simulink library "commutil"  (Simulink 5.0)
values from neighbouring files (symbols this model uses):
  En = get_param(block, 'maskenables')    [commblkawgnchan.m]    (also in commblkbernoullisrc.m; commblkdemap.m; commblkdrpt.m; commblkeyescatdisc.m = get_param(block, 'MaskEnables'))
  IPValues = (0:M-1)    [commblkdemap.m]    (also in commblkmap.m)
  OPValues = MapVec    [commblkdemap.m]    (also in commblkmap.m)
undefined symbols (not defined in the file or in its folder): SatValue
libraries: commutil x8, dsparch2 x1, dspswit2 x1
settings Model: RequirementInfo=9  Creator=tdelve  LastModifiedBy=mmclerno

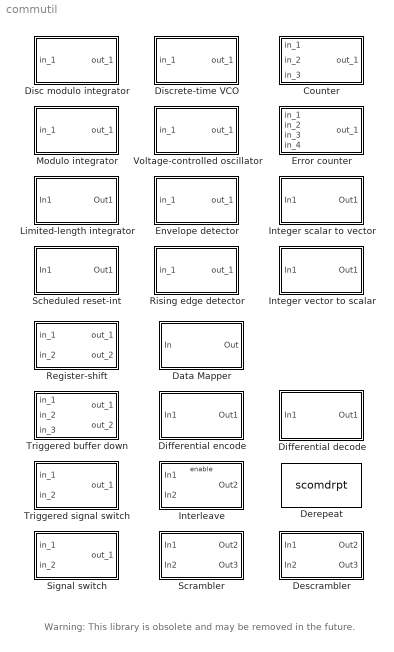
== system commutil ==
  note: Warning:  This library is obsolete and may be
      | removed in the future.
  Counter : Subsystem  mask(Resettable number counter){thld=.2}
      mask prompts: thld "Threshold:"
      mask help: If the 1st inport value is larger than the threshold, the counter increases one at the rising edge of the 2nd inport pulse.
      mask Help: If the signal at the 1st inport is larger than or equal to the given threshold at the rising edge of the 2nd inport, the counter increases by one. The rising edge of the 3rd port resets the counter to zero.
      mask Display:
      | plot(0,0,100,100,[5 10 10 8 10 12 10 10 15],[5 5 12 8 12 8 12 15 15]+40,[5 10 10 8 10 12 10 10 15],[5 5 12 8 12 8 12 15 15]);
      | disp('Counter')
  Data Mapper : Subsystem  mask(Data Mapper){MapMode=Binary to Gray, M=8, MapVec=[0 1 3 2 7 6 4 5]}
      mask prompts: MapMode "Mapping mode:"; M "Symbol set size (M):"; MapVec "Mapping vector:"
      mask help: Map integer symbols from one coding scheme to another.
      mask init:
      | [En,IPValues,OPValues,SatValue]=commblkmapdata(gcb,'init',{MapMode M MapVec});
      mask Help:
      | <P><FONT SIZE=+0>The Data Mapper block accepts integer inputs and produces
      | integer outputs. You can select one of four mapping modes: <B>Binary to
      | Gray, Gray to Binary, User Defined, or Straight Through</B>.</FONT>
      | 
      | <P><FONT SIZE=+0>Gray coding is an ordering of binary numbers such that
      | all adjacent numbers differ by only one bit. However, the inputs and outputs
      | of this block are integers, not binary vectors. As a result, the first
      | two mapping modes perform code conversions as follows:</FONT>
      | <UL type="disc">
      | <LI>
      | <FONT SIZE=+0>In the <B>Binary to Gray</B> mode, the output from this block
      | is the integer equivalent of the Gray code bit representation for the input
      | integer.</FONT></LI>
      | 
      | <LI>
      | <FONT SIZE=+0>In the <B>Gray to Binary</B> mode, the output from this block
      | is the integer position of the binary equivalent of the input integer in
      | a Gray code ordering.</FONT></LI>
      | </UL>
      | <FONT SIZE=+0>As an example, the table below shows both the <B>Binary to
      | Gray</B> and <B>Gray to Binary</B> mappings for integers in the range 0
      | to 7.</FONT>
      | <BR>&nbsp;
      | <TABLE BORDER CELLPADDING=9 WIDTH="480" >
      | <TR>
      | <TD COLSPAN="4"><B><FONT SIZE=+0>Table 1: Example of Binary to Gray and
      | Gray to Binary Mappings</FONT></B></TD>
      | </TR>
      | 
      | <TR>
      | <TD COLSPAN="2" WIDTH="50%">
      | <CENTER><B><FONT SIZE=+0>Binary to Gray Mode</FONT></B></CENTER>
      | </TD>
      | 
      | <TD COLSPAN="2" WIDTH="50%">
      | <CENTER><B><FONT SIZE=+0>Gray to Binary Mode</FONT></B></CENTER>
      | </TD>
      | </TR>
      | 
      | <TR>
      | <TD WIDTH="25%">
      | <CENTER><B><FONT SIZE=+0>Input</FONT></B></CENTER>
      | </TD>
      | 
      | <TD WIDTH="25%">
      | <CENTER><B><FONT SIZE=+0>Output</FONT></B></CENTER>
      | </TD>
      | 
      | <TD WIDTH="25%">
      | <CENTER><B><FONT SIZE=+0>Input</FONT></B></CENTER>
      | </TD>
      | 
      | <TD WIDTH="25%">
      | <CENTER><B><FONT SIZE=+0>Output</FONT></B></CENTER>
      | </TD>
      | </TR>
      | 
      | <TR>
      | <TD WIDTH="25%">
      | <CENTER><FONT SIZE=+0>0</FONT></CENTER>
      | </TD>
      | 
      | <TD WIDTH="25%">
      | <CENTER><FONT SIZE=+0>0 <I>(000)</I></FONT></CENTER>
      | </TD>
      | 
      | <TD WIDTH="25%">
      | <CENTER><FONT SIZE=+0>0 <I>(000)</I></FONT></CENTER>
      | </TD>
      | 
      | <TD WIDTH="25%">
      | <CENTER><FONT SIZE=+0>0</FONT></CENTER>
      | </TD>
      | </TR>
      | 
      | <TR>
      | <TD WIDTH="25%">
      | <CENTER><FONT SIZE=+0>1</FONT></CENTER>
      | </TD>
      | 
      | <TD WIDTH="25%">
      | <CENTER><FONT SIZE=+0>1 <I>(001)</I></FONT></CENTER>
      | </TD>
      | 
      | <TD WIDTH="25%">
      | <CENTER><FONT SIZE=+0>1 <I>(001)</I></FONT></CENTER>
      | </TD>
      | 
      | <TD WIDTH="25%">
      | <CENTER><FONT SIZE=+0>1</FONT></CENTER>
      | </TD>
      | </TR>
      | 
      | <TR>
      | <TD WIDTH="25%">
      | <CENTER><FONT SIZE=+0>2</FONT></CENTER>
      | </TD>
      | 
      | <TD WIDTH="25%">
      | <CENTER><FONT SIZE=+0>3 <I>(011)</I></FONT></CENTER>
      | </TD>
      | 
      | <TD WIDTH="25%">
      | <CENTER><FONT SIZE=+0>2 <I>(010)</I></FONT></CENTER>
      | </TD>
      | 
      | <TD WIDTH="25%">
      | <CENTER><FONT SIZE=+0>3</FONT></CENTER>
      | </TD>
      | </TR>
      | 
      | <TR>
      | <TD WIDTH="25%">
      | <CENTER><FONT SIZE=+0>3</FONT></CENTER>
      | </TD>
      | 
      | <TD WIDTH="25%">
      | <CENTER><FONT SIZE=+0>2 <I>(010)</I></FONT></CENTER>
      | </TD>
      | 
      | <TD WIDTH="25%">
      | <CENTER><FONT SIZE=+0>3 <I>(011)</I></FONT></CENTER>
      | </TD>
      | 
      | <TD WIDTH="25%">
      | <CENTER><FONT SIZE=+0>2</FONT></CENTER>
      | </TD>
      | </TR>
      | 
      | <TR>
      | <TD WIDTH="25%">
      | <CENTER><FONT SIZE=+0>4</FONT></CENTER>
      | </TD>
      | 
      | <TD WIDTH="25%">
      | <CENTER><FONT SIZE=+0>6 <I>(110)</I></FONT></CENTER>
      | </TD>
      | 
      | <TD WIDTH="25%">
      | <CENTER><FONT SIZE=+0>4 <I>(100)</I></FONT></CENTER>
      | </TD>
      | 
      | <TD WIDTH="25%">
      | <CENTER><FONT SIZE=+0>7</FONT></CENTER>
      | </TD>
      | </TR>
      | 
      | <TR>
      | <TD WIDTH="25%">
      | <CENTER><FONT SIZE=+0>5</FONT></CENTER>
      | </TD>
      | 
      | <TD WIDTH="25%">
      | <CENTER><FONT SIZE=+0>7 <I>(111)</I></FONT></CENTER>
      | </TD>
      | 
      | <TD WIDTH="25%">
      | <CENTER><FONT SIZE=+0>5 <I>(101)</I></FONT></CENTER>
      | </TD>
      | 
      | <TD WIDTH="25%">
      | <CENTER><FONT SIZE=+0>6</FONT></CENTER>
      | </TD>
      | </TR>
      | 
      | <TR>
      | <TD WIDTH="25%">
      | <CENTER><FONT SIZE=+0>6</FONT></CENTER>
      | </TD>
      | 
      | <TD WIDTH="25%">
      | <CENTER><FONT SIZE=+0>5 <I>(101)</I></FONT></CENTER>
      | </TD>
      | 
      | <TD WIDTH="25%">
      | <CENTER><FONT SIZE=+0>6 <I>(110)</I></FONT></CENTER>
      | </TD>
      | 
      | <TD WIDTH="25%">
      | <CENTER><FONT SIZE=+0>4</FONT></CENTER>
      | </TD>
      | </TR>
      | 
      | <TR>
      | <TD WIDTH="25%">
      | <CENTER><FONT SIZE=+0>7</FONT></CENTER>
      | </TD>
      | 
      | <TD WIDTH="25%">
      | <CENTER><FONT SIZE=+0>4 <I>(100)</I></FONT></CENTER>
      | </TD>
      | 
      | <TD WIDTH="25%">
      | <CENTER><FONT SIZE=+0>7 <I>(111)</I></FONT></CENTER>
      | </TD>
      | 
      | <TD WIDTH="25%">
      | <CENTER><FONT SIZE=+0>5</FONT></CENTER>
      | </TD>
      | </TR>
      | </TABLE>
      | <FONT SIZE=+0></FONT>
      | 
      | <P><FONT SIZE=+0>When you select the <B>User Defined</B> mode, you can
      | use any arbitrary mapping by providing a vector to specify the output ordering.
      | For example, the vector <NOBR>[1</NOBR></FONT><NOBR> <FONT SIZE=+0>5 0
      | 4 2 7 3 6]</FONT></NOBR><FONT SIZE=+0> defines the following mapping:</FONT>
      | <UL>
      | <LI>
      | <FONT SIZE=+0>0 - 1</FONT></LI>
      | 
      | <LI>
      | <FONT SIZE=+0>1 - 5</FONT></LI>
      | 
      | <LI>
      | <FONT SIZE=+0>2 - 0</FONT></LI>
      | 
      | <LI>
      | <FONT SIZE=+0>3 - 4</FONT></LI>
      | 
      | <LI>
      | <FONT SIZE=+0>4 - 2</FONT></LI>
      | 
      | <LI>
      | <FONT SIZE=+0>5 - 7</FONT></LI>
      | 
      | <LI>
      | <FONT SIZE=+0>6 - 3</FONT></LI>
      | 
      | <LI>
      | <FONT SIZE=+0>7 - 6</FONT></LI>
      | </UL>
      | <FONT SIZE=+0>When you select the <B>Straight Through</B> mode, the output
      | is equal to the input.</FONT>
      mask StyleString: popup(Binary to Gray|Gray to Binary|User Defined|Straight through),edit,edit
      mask CallbackString: commblkmapdata(gcb,'MapMode');||
      mask Display: disp('Data\nMapper');
  Derepeat : S-Function  FunctionName=scomdrpt  Parameters=N,ic,frame,nchans,mode  mask(Derepeat){N=10, ic=0, frame=off, nchans=1, mode=Maintain input frame size}
      mask prompts: N "Derepeat factor, N:"; ic "Initial condition:"; frame "Frame-based inputs"; nchans "Number of channels:"; mode "Framing:"
      mask help: Derepeat by an integer factor. The value of each output sample is the mean value of N consecutive input samples.
      mask init:
      | commblkdrpt(gcb,'init');
      mask Help: web(commbhelp);
      mask StyleString: edit,edit,checkbox,edit,popup(Maintain input frame size|Maintain input frame rate)
      mask CallbackString: ||commblkdrpt(gcb,'cbFBFlag');||commblkdrpt(gcb,'cbMode');
      mask Display: disp(sprintf('Derepeat\n/%d',N));
  Descrambler : Subsystem  mask(Descrambler){M=2, poly=[0 -5 -6], ini_sta=[1 1 0 1 0 1]}
      mask prompts: M "Calculation base:"; poly "Scramble polynomial:"; ini_sta "Initial states"
      mask help: This block outputs the descrambled signal of the 1st inport input symbol. The block input and output are controlled by the rising edge of the 2nd inport input signal. The block works only if the enable signal is on. This block takes scalar input only. The second output port outputs the states of the registers.
      mask init:
      | if M<=0, error('Scramble calculation base must be a positive interger.'); end
      | if max(poly)>=M
      |  error('Scramble polynomial coefficients must be less than calculation base.');
      | elseif min(poly)<0
      |   tmp = zeros(1, abs(min(poly))+1);
      |   for i = 1:length(poly), tmp(abs(poly(i))+1) = 1; end
      |   poly = tmp;
      | end
      | if poly(1) == 0, poly(1) = 1; end
      | s = length(poly)-1;
      mask Help: Scrambling is a simple method to minimize transferring a long series of the same number, such as 1 or 0. Its operation is based on a scrambler polynomial g(x). This block descrambles the input signal using the polynomial g(x). You can specify the polynomial using the coefficients of the polynomial or by specifying the terms for which the coefficient is 1; for other terms, the coefficient is the default, 0. For example g = [1 0 0 0 0 0 1 0 1] and g = [0 -6 -8] represent the same polynomial g(x) = 1 + x^(-6) + x^(-8). The initial state of at least one of the registers must be nonzero in order to generate a nonzero sequence. The Descrambler block inherits the sample time from the block that inputs to it.
      mask Display:
      | disp('Descrambler')
      | plot(0,0,100,100,[5 10 10 8 10 12 10 10 15],[5 5 12 8 12 8 12 15 15]+10)
  Differential decode : Subsystem  mask(Binary differential decoder){td=1}
      mask prompts: td "Symbol interval (sec):"
      mask help: The binary scalar output of this block, D(k), is a logical differential computation of the binary scalar input of this block, M(k). D(k) = rem(M(k) + M(k-1) + 1,2).
      mask Help: This block decodes a differential encoded signal. Let the input signal be M(k) and the output signal be D(k). Then, D(k) = rem(M(k) + M(k-1) + 1,2), where M(k-1) is the previous input to this block. The time interval between M(k) and M(k-1) is td, the symbol interval.
      mask Display: disp('Differential\ndecoder')
  Differential encode : Subsystem  mask(Binary differential encoder){td=1}
      mask prompts: td "Symbol interval (sec):"
      mask help: The binary scalar output of this block, D(k), is a logical differential computation of the binary scalar input to this block, M(k) with the previous output of this block D(k-1). D(k) = rem(M(k) + D(k-1),2)
      mask Help: This block encodes the binary scalar signal using the differential encode method. Let the input signal be M(k) and the output signal be D(k). Then, D(k) = rem(M(k) + D(k-1),2), where D(k-1) is the previous output of this block. The time interval between D(k) and D(k-1) is td, the symbol interval.
      mask Display: disp('Differential\nencoder')
  Disc modulo integrator : Subsystem  mask(Discrete-time modulo integrator){modu=1, init=0, ts=.01}
      mask prompts: modu "Modulo bound:"; init "Initial state:"; ts "Sample time (sec):"
      mask help: When the absolute value of the state exceeds the modulo bound, the state is reset to be the remainder of the state divided by the modulo bound.
      mask Help: This block calculate the integration of the input signal. The absolute value of this integrator will not exceed the specified module bound. The state value is reset to be the remainder of the state divided by the modulo bound. This block can only be used for scale value calculation. This block is a discrete-time integration block.
      mask Display: disp('Discrete\nmod-int')
  Discrete-time VCO : Subsystem  mask(Voltage-controlled oscillator){Ac=1, Fc=10, Kc=1, Ph=0, ts=.01}
      mask prompts: Ac "Output amplitude:"; Fc "Oscillation frequency (Hz):"; Kc "Input sensitivity:"; Ph "Initial phase (rad):"; ts "Sample time (sec):"
      mask help: The frequency of the output signal changes with the input signal.
      mask init:
      | pi2=2*pi;Kc=Kc*pi2*ts(1);Fc=Fc*pi2;
      mask Help: This block causes the frequency of the sinusoidal oscillation signal to change with the input signal voltage. The input sensitivity is the preamplifier added to the input signal. This block uses a discrete-time integrator.
      mask Display: disp('Discrete\nVCO')
  Envelope detector : Subsystem  mask(Envelope detector){x='upper'}
      mask prompts: x "Boundary side ('upper' or 'lower'):"
      mask help: Output the upper or lower boundary of the input signal.
      mask init:
      | if length(x)<2, error('Error in Envelop Detector');end;x=x(1:2);g=1;if x=='lo', g=-1;end;
      mask Help: This block detects the upper or lower boundary of the envelope of the input signal. This block finds the maximum or minimum value of the input signal. The block is noise sensitive.
      mask Display: disp('Envelope\ndetector')
  Error counter : Subsystem  mask(Error counter){thld=0.2, tol=eps}
      mask prompts: thld "Threshold:"; tol "Tolerance:"
      mask help: If the 1st and 2nd inport values do not match at the rising edge of the 3rd inport, the counter increases by one.
      mask Help: If the signals at the 1st and 2nd inport do not match at the rising edge of the 3rd inport pulse, the counter increases by one. The rising edge of the 4th inport resets the counter to zero.
      mask Display:
      | plot(0,0,100,100,[5 10 10 8 10 12 10 10 15],[5 5 12 8 12 8 12 15 15]+30,[5 10 10 8 10 12 10 10 15],[5 5 12 8 12 8 12 15 15]);
      | disp('Err count')
  Integer scalar to vector : Subsystem  mask(Decimal to base M vector){len=4, p=2, MSBFlag=off}
      mask prompts: len "Output vector length:"; p "Conversion base M:"; MSBFlag "First element of output vector is most significant digit"
      mask help: Convert decimal integer input to base M integer and output each position of the converted integer using output vector.
      mask Help:
      | This block converts decimal integer scalar input to a base M integer. M must be a positive integer. The block outputs the base M integer using a vector. The 1st element in the output vector contains the 1's position. The 2nd element in the output vector contains the M's position, and so on. The output vector length is given by setting the parameter entry.
      | 
      | The most significant digit may be output as the first element of the vector by selecting the check box.
      mask Display: disp('Sca to vec\nconverter')
  Integer vector to scalar : Subsystem  mask(Base M vector to decimal integer){p=2, MSBFlag=off}
      mask prompts: p "Input integer base M:"; MSBFlag "First element of input vector is most significant digit"
      mask help: Convert base M integer with each position in the input vector into scalar decimal output.
      mask Help:
      | This block convert the base M vector into scalar decimal integer output. Each element of the input vector is one position of the digit of the base M integer. The 1st element in the input vector contains the 1's position. The 2nd element in the input vector contains the M's position.
      | 
      | The first element of the input vector may be used as the most significant digit by selecting the check box.
      mask Display: disp('Vec to sca\nconverter')
  Interleave : Subsystem  TreatAsAtomicUnit=on  mask(Block Interleave){N=3, M=4}
      mask prompts: N "Input code row length (N):"; M "Interleave row number (M):"
      mask help: This block takes a new symbol from the 1st input port and outputs an interleaved signal to the 1st output port at the rising edge of the 2nd inport input signal. The block works only if the enable signal is on. This block takes scalar input only. The output is the interleaved result.
      mask init:
      | if N<=0, error('Row length must be a positive number.'); end;
      | if M<=0 error('Interleave row number must be a positive number.'); end;
      mask Help: Block interleaving is a simple method to convert burst errors to random errors. The block keeps an N-column by M-row buffer. The input to the buffer is row by row. The output from this buffer is column by column. The output of this block has an N*M step delay from the starting point of the input. Before a meaningful message is output, this block outputs 0s. Block deinterleave uses the Block Interleave function block. Note that the column and row number assignments for block deinterleave should be the exact reverse of block interleave. Block deinterleave works only when the enable signal is on.
      mask Display:
      | disp('Block\ninterleave')
      | plot(0,0,100,100,[5 10 10 8 10 12 10 10 15],[5 5 12 8 12 8 12 15 15]+10)
  Limited-length integrator : Subsystem  mask(Windowed integration){vec=2, T=1, sample_time=.1, method='first order'}
      mask prompts: vec "Input vector size:"; T "Integration window length:"; sample_time "Sample time (sec):"; method "Method ('forward', 'backward', or 'first order'):"
      mask help: Output the integration of the input from time t-T to t, where T is the size of the integration window.
      mask Help: This block outputs\n t\n int u(t) dt\n t-T\n The output vector length is the same as the input vector length. You can choose forward, backward, or first order integration methods.
      mask Display: disp('Windowed\nintegrator')
  Modulo integrator : Subsystem  mask(Modulo integrator){modu=1, init=0}
      mask prompts: modu "Modulo bound:"; init "Initial state:"
      mask help: When the absolute value of the state exceeds the modulo bound, the state is reset to be the remainder of the state divided by the modulo bound.
      mask Help: This block calculate the integration of the input signal. The absolute value of this integrator will not exceed the specified module bound. The state value is reset to be the remainder of the state divided by the modulo bound. This block can only be used for scale value calculation. This block is a continuous-time integration block.
      mask Display: disp('Modulo\nintegrator')
  Register-shift : Subsystem  mask(Register-shift){shft_out=[127:-1:0], thrhld=.1}
      mask prompts: shft_out "Delay steps (output length is same as this vector size):"; thrhld "Threshold in detecting the rising edge of the pulse:"
      mask help: The rising edge of the 2nd port pulse triggers the block to input the 1st port data and to shift the register.
      mask init:
      | len_rg=length(shft_out);
      mask Help: This block stores the scalar input signal from the 1st input port at the rising edge of the pulse from the 2nd port. The 1st outport outputs a vector with its size the same as the "Delay steps" entree of this block. The maximum delay is the register size of this block. The second outport outputs a positive pulse when the register is\nrefreshed.
      mask Display:
      | plot(0,0,100,100,[5 10 10 8 10 12 10 10 15],[5 5 12 8 12 8 12 15 15]+10,[5 10 10 8 10 12 10 10 15]+80,[5 5 12 8 12 8 12 15 15]+10);
      | disp('Reg. shift')
  Rising edge detector : Subsystem  mask(Edge detection){thld=0.5}
      mask prompts: thld "Threshold:"
      mask help: Detect the rising edge of the input signal. Output one when the rising edge is detected.
      mask Help: This block outputs one when the input signal reaches a value larger than or equal to the given threshold value at the current time and the value was below the threshold one time step before. Otherwise, the block outputs zero.
      mask Display: plot(0,0,100,100,[5 10 10 8 10 12 10 10 15]+80,[5 5 12 8 12 8 12 15 15]+35, [5 10 10 15 15 20]-5,[5 5 10 10 5 5]+40);disp('Edge det.')
  Scheduled reset-int : Subsystem  mask(Scheduled reset integration){td=Inf, ts=.05, limit=2}
      mask prompts: td "Scheduled reset time interval and offset (sec):"; ts "Computation sample time and offset (sec):"; limit "Modulo bound:"
      mask help: Reset the state to be zero(s) at the scheduled reset sample point.
      mask Help: This block resets the state(s) to be zero(s) at the reset time points. The reset interval can be a two-element vector with the second element as offset. The computation sample time must be smaller than the reset interval. The block resets the state value to be the remainder of the state divided by the modulo bound when the absolute value of the state is larger than the modulo bound.
      mask Display: disp('Scheduled\nreset-int')
  Scrambler : Subsystem  mask(Scrambler){M=2, poly=[0 -5 -6], ini_sta=[1 1 0 1 0 1]}
      mask prompts: M "Calculation base:"; poly "Scramble polynomial:"; ini_sta "Initial states"
      mask help: This block outputs the scrambled signal of the 1st inport input symbol. The block input and output are controlled by the rising edge of the 2nd inport input signal. This block takes scalar input only. The first output port outputs the scrambled signal. The second output port outputs the states of the registers.
      mask init: same as commutil/Descrambler
      mask Help: Scrambling is a simple method to minimize transferring a long series of the same number, such as 1 or 0. Its operation is based on a scrambler polynomial g(x). This block scrambles the input signal using the polynomial g(x). You can specify the polynomial using the coefficients of the polynomial or by specifying the terms for which the coefficient is 1; for other terms, the coefficient is the default, 0. For example g = [1 0 0 0 0 0 1 0 1] and g = [0 -6 -8] represent the same polynomial g(x) = 1 + x^(-6) + x^(-8). The initial state of at least one of the registers must be nonzero in order to generate a nonzero sequence. The Scrambler block inherits the sample time from the block that inputs to it.
      mask Display:
      | disp('Scrambler')
      | plot(0,0,100,100,[5 10 10 8 10 12 10 10 15],[5 5 12 8 12 8 12 15 15]+10)
  Signal switch : Subsystem  mask(Vector signal re-distribution){sw=[1 2;2 3;3 1], df=[0 0]}
      mask prompts: sw "Switch box (column number equals block output length):"; df "Default value:"
      mask help: The output distribution pattern follows the ith row of the switch box, where i is the input from the second port.
      mask Help: This block follows the switch pattern of ith row in the switch box when the second input port has value i.  When the value in the second input is larger than the switch box row number or less than 1, the block outputs the defualt value.
      mask Display: disp('Switch\nbox')
  Triggered buffer down : Subsystem  mask(Triggered buffer down){in_size=128, ini_idx=[0 0 0], idx_inc=[1 2 3], thrshld=.1, cycl_flag=1}
      mask prompts: in_size "Input signal vector size:"; ini_idx "Initial index (integer vector):"; idx_inc "Increment for each index (integer vector):"; thrshld "Trigger threshold:"; cycl_flag "When index exceed register size, 1: cyclic out, 0: zero out:"
      mask help: Rising edge of the 2nd port triggers 1st port vector signal in. Rising edge of the 3rd port triggers 1st outport signal out.
      mask init:
      | out_size=length(ini_idx);
      mask Help: The block refreshes its registers with the vector input from the 1st inport at the rising edge of the 2nd inport pulse. The 1st outport outputs the elements of the registers starting with the given initial index. The rising edge of the 3rd inport pulse triggers the 1st output to output the register value with the index increasing the increment value. The second outport outputs a spike pulse when the internal register is refreshed.
      mask Display:
      | plot(0,0,100,100,[5 10 10 8 10 12 10 10 15]-5,[5 5 12 8 12 8 12 15 15],[5 10 10 8 10 12 10 10 15]-5,[5 5 12 8 12 8 12 15 15]+45);
      | disp('Buffer dwn')
  Triggered signal switch : Subsystem  mask(Vector signal re-distribution){sw=[1 2 3;2 3 1;3 1 2], ke=[-1 -1 -1], in=[0 0 0], tt=.1}
      mask prompts: sw "Switch box (column number equals block output length):"; ke "Keeping value (flag 0 element in switch box):"; in "Initial value (before the 1st trigger is detected):"; tt "Trigger threshold:"
      mask help: The rising edge from the 2nd inport triggers the block to output the input element with the index given in the next row of the switch box.
      mask Help: When current switch box row is [i,j], the 1st and 2nd elements output the ith and jth input respectively. The switch_box column number must be same lengths as the output, keep_value, and init_value. The rising edge of the 2nd inport triggers the distribution pattern following the next row of the switch_box. With 0 element in switch_box, the output keeps the last output value with a >=0 keep_value; it equals init_val otherwise.
      mask Display: plot(0,0,100,100,[5 10 10 8 10 12 10 10 15],[5 5 12 8 12 8 12 15 15]);disp('Vct re-arr')
  Voltage-controlled oscillator : Subsystem  mask(Voltage-controlled oscillator){Ac=1, Fc=10, Kc=1, Ph=0}
      mask prompts: Ac "Output amplitude:"; Fc "Oscillation frequency (Hz):"; Kc "Input sensitivity:"; Ph "Initial phase (rad):"
      mask help: The frequency of the output signal changes with the input signal.
      mask init:
      | pi2=2*pi;
      mask Help: This block causes the frequency of the sinusoidal oscillation signal to change with the input signal voltage. The input sensitivity is the preamplifier added to the input signal.
      mask Display: disp('VCO')

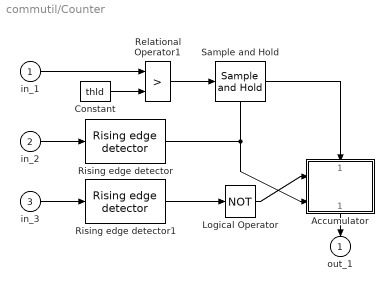
== system commutil/Counter ==
  in_1 : Inport
  in_2 : Inport  Port=2
  in_3 : Inport  Port=3
  Accumulator : Subsystem  Orientation=down  TreatAsAtomicUnit=on
  Constant : Constant  Value=thld
  Logical Operator : Logic  Operator=NOT
  Relational Operator1 : RelationalOperator  Operator=>  InputSameDT=on
  Rising edge detector : commutil/Rising edge detector  thld=0.5
  Rising edge detector1 : commutil/Rising edge detector  thld=0.5
  Sample and Hold : dspswit2/Sample and Hold  trig=Rising edge  initCond=0
  out_1 : Outport  Orientation=down  InitialOutput=0
  wires:
  Accumulator/1("  ") -> out_1/1
  Sample and Hold/1 -> Accumulator/1(" ")
  Rising edge detector/1 -> Accumulator/Trigger, Sample and Hold/Trigger
  in_2/1 -> Rising edge detector/1
  Rising edge detector1/1 -> Logical Operator/1
  in_3/1 -> Rising edge detector1/1
  Constant/1 -> Relational Operator1/2
  in_1/1 -> Relational Operator1/1
  Relational Operator1/1 -> Sample and Hold/1
  Logical Operator/1 -> Accumulator/Enable

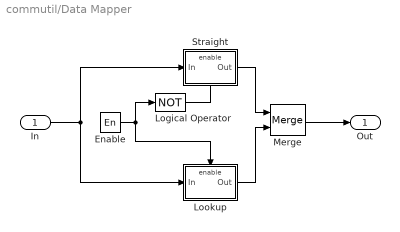
== system commutil/Data Mapper ==
  In : Inport
  Enable : Constant  Value=En
  Logical Operator : Logic  Operator=NOT  Inputs=1
  Lookup : Subsystem  TreatAsAtomicUnit=on
  Merge : Merge
  Straight : Subsystem  TreatAsAtomicUnit=on
  Out : Outport
  wires:
  Straight/1(Out) -> Merge/1
  In/1 -> Straight/1(In), Lookup/1(In)
  Lookup/1(Out) -> Merge/2
  Merge/1 -> Out/1
  Logical Operator/1 -> Straight/Enable
  Enable/1 -> Logical Operator/1, Lookup/Enable

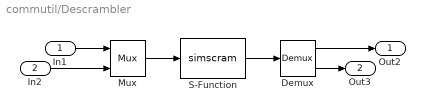
== system commutil/Descrambler ==
  In1 : Inport
  In2 : Inport  Port=2
  Demux : Demux  Outputs=[1 s]
  Mux : Mux  Inputs=2
  S-Function : S-Function  FunctionName=simscram  Parameters=M, poly, 1, ini_sta
  Out2 : Outport  InitialOutput=0
  Out3 : Outport  Port=2  InitialOutput=0
  wires:
  S-Function/1 -> Demux/1
  Mux/1 -> S-Function/1
  In2/1 -> Mux/2
  In1/1 -> Mux/1
  Demux/2 -> Out3/1
  Demux/1 -> Out2/1

== system commutil/Differential decode ==
  In1 : Inport
  Logical Operator : Logic  Operator=XOR
  Logical Operator1 : Logic  Operator=NOT  Inputs=1
  Unit Delay : UnitDelay  SampleTime=td
  Out1 : Outport  InitialOutput=0
  wires:
  Logical Operator1/1 -> Out1/1
  Unit Delay/1 -> Logical Operator/2
  In1/1 -> Logical Operator/1, Unit Delay/1
  Logical Operator/1 -> Logical Operator1/1

== system commutil/Differential encode ==
  In1 : Inport
  Logical Operator : Logic  Operator=XOR
  Logical Operator1 : Logic  Operator=NOT  Inputs=1
  Unit Delay : UnitDelay  Orientation=left  SampleTime=td
  Out1 : Outport  InitialOutput=0
  wires:
  In1/1 -> Logical Operator/1
  Unit Delay/1 -> Logical Operator/2
  Logical Operator1/1 -> Unit Delay/1, Out1/1
  Logical Operator/1 -> Logical Operator1/1

== system commutil/Disc modulo integrator ==
  in_1 : Inport
  Gain1 : Gain  Gain=ts(1)  SaturateOnIntegerOverflow=on
  Sum : Sum  SaturateOnIntegerOverflow=on  InputSameDT=on
  Unit Delay : UnitDelay  X0=init  SampleTime=ts
  module : Fcn  Expr=rem(u[1],modu)
  out_1 : Outport  InitialOutput=0
  wires:
  Sum/1 -> module/1
  in_1/1 -> Gain1/1
  Gain1/1 -> Sum/1
  module/1 -> Unit Delay/1
  Unit Delay/1 -> Sum/2, out_1/1

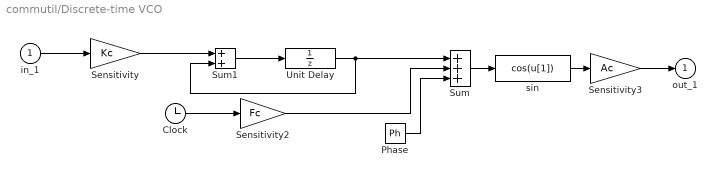
== system commutil/Discrete-time VCO ==
  in_1 : Inport
  Clock : Clock
      settings: Decimation=10
  Phase : Constant  Value=Ph
  Sensitivity : Gain  Gain=Kc  SaturateOnIntegerOverflow=on
  Sensitivity2 : Gain  Gain=Fc  SaturateOnIntegerOverflow=on
  Sensitivity3 : Gain  Gain=Ac  SaturateOnIntegerOverflow=on
  Sum : Sum  Inputs=+++  SaturateOnIntegerOverflow=on  InputSameDT=on
  Sum1 : Sum  SaturateOnIntegerOverflow=on  InputSameDT=on
  Unit Delay : UnitDelay  SampleTime=ts
  sin : Fcn  Expr=cos(u[1])
  out_1 : Outport  InitialOutput=0
  wires:
  in_1/1 -> Sensitivity/1
  Sensitivity/1 -> Sum1/1
  Sum1/1 -> Unit Delay/1
  Sum/1 -> sin/1
  Clock/1 -> Sensitivity2/1
  Sensitivity2/1 -> Sum/2
  Unit Delay/1 -> Sum1/2, Sum/1
  Phase/1 -> Sum/3
  sin/1 -> Sensitivity3/1
  Sensitivity3/1 -> out_1/1

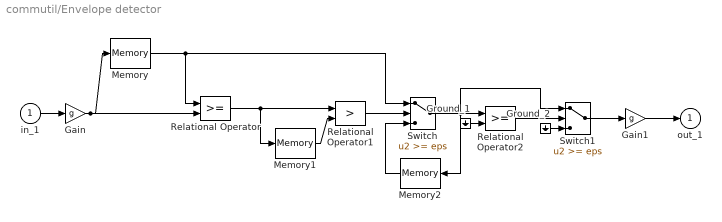
== system commutil/Envelope detector ==
  in_1 : Inport
  Gain : Gain  Gain=g  SaturateOnIntegerOverflow=on
  Gain1 : Gain  Gain=g  SaturateOnIntegerOverflow=on
  Ground_1 : Ground
  Ground_2 : Ground
  Memory : Memory
  Memory1 : Memory
  Memory2 : Memory  Orientation=left
  Relational Operator : RelationalOperator  InputSameDT=on
  Relational Operator1 : RelationalOperator  Operator=>  InputSameDT=on
  Relational Operator2 : RelationalOperator  InputSameDT=on
  Switch : Switch  Threshold=eps  SaturateOnIntegerOverflow=on  InputSameDT=on
  Switch1 : Switch  Threshold=eps  SaturateOnIntegerOverflow=on  InputSameDT=on
  out_1 : Outport  InitialOutput=0
  wires:
  Ground_2/1 -> Switch1/3
  Ground_1/1 -> Relational Operator2/2
  Switch/1 -> Switch1/1, Relational Operator2/1, Memory2/1
  Relational Operator2/1 -> Switch1/2
  Switch1/1 -> Gain1/1
  Memory/1 -> Switch/1, Relational Operator/1
  Memory1/1 -> Relational Operator1/2
  Relational Operator/1 -> Relational Operator1/1, Memory1/1
  Relational Operator1/1 -> Switch/2
  Memory2/1 -> Switch/3
  in_1/1 -> Gain/1
  Gain/1 -> Relational Operator/2, Memory/1
  Gain1/1 -> out_1/1

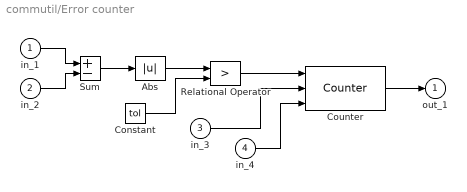
== system commutil/Error counter ==
  in_1 : Inport
  in_2 : Inport  Port=2
  in_3 : Inport  Port=3
  in_4 : Inport  Port=4
  Abs : Abs  SaturateOnIntegerOverflow=on
  Constant : Constant  Value=tol
  Counter : commutil/Counter  thld=.2
  Relational Operator : RelationalOperator  Operator=>  InputSameDT=on
  Sum : Sum  Inputs=+-  SaturateOnIntegerOverflow=on  InputSameDT=on
  out_1 : Outport  InitialOutput=0
  wires:
  Constant/1 -> Relational Operator/2
  Abs/1 -> Relational Operator/1
  Sum/1 -> Abs/1
  in_2/1 -> Sum/2
  in_1/1 -> Sum/1
  Counter/1 -> out_1/1
  in_3/1 -> Counter/2
  Relational Operator/1 -> Counter/1
  in_4/1 -> Counter/3

== system commutil/Integer scalar to vector ==
  In1 : Inport
  Integer scalar to vector : S-Function  FunctionName=scomsc2vec  Parameters=len, p, MSBFlag
  Out1 : Outport  InitialOutput=0
  wires:
  Integer scalar to vector/1 -> Out1/1
  In1/1 -> Integer scalar to vector/1

== system commutil/Integer vector to scalar ==
  In1 : Inport
  Integer vector to scalar : S-Function  FunctionName=scomvec2sc  Parameters=p,MSBFlag
  Out1 : Outport  InitialOutput=0
  wires:
  Integer vector to scalar/1 -> Out1/1
  In1/1 -> Integer vector to scalar/1

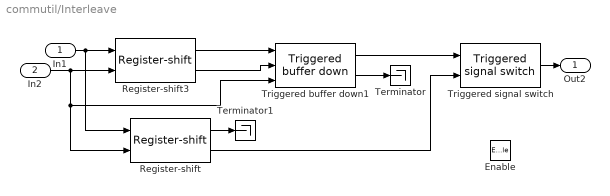
== system commutil/Interleave ==
  In1 : Inport
  In2 : Inport  Port=2
  Enable : EnablePort
  Register-shift : commutil/Register-shift  shft_out=[M:-1:1]  thrhld=.1
  Register-shift3 : commutil/Register-shift  shft_out=[N*M:-1:1]  thrhld=.1
  Terminator : Terminator
  Terminator1 : Terminator
  Triggered buffer down1 : commutil/Triggered buffer down  in_size=N*M  ini_idx=[0:N-1]  idx_inc=N*ones(1,N)  thrshld=.1  cycl_flag=1
  Triggered signal switch : commutil/Triggered signal switch  sw=[1:N]'  ke=-1  in=0  tt=.1
  Out2 : Outport  InitialOutput=0
  wires:
  Register-shift/2 -> Triggered signal switch/2
  Register-shift/1 -> Terminator1/1
  Triggered buffer down1/1 -> Triggered signal switch/1
  Triggered signal switch/1 -> Out2/1
  Register-shift3/2 -> Triggered buffer down1/2
  Register-shift3/1 -> Triggered buffer down1/1
  Triggered buffer down1/2 -> Terminator/1
  In2/1 -> Register-shift3/2, Register-shift/2, Triggered buffer down1/3
  In1/1 -> Register-shift3/1, Register-shift/1

== system commutil/Limited-length integrator ==
  In1 : Inport
  Limited-length integrator : S-Function  FunctionName=moveint  Parameters=vec,T,sample_time,method
  Out1 : Outport  InitialOutput=0
  wires:
  In1/1 -> Limited-length integrator/1
  Limited-length integrator/1 -> Out1/1

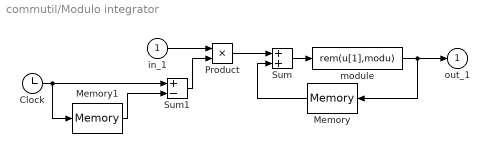
== system commutil/Modulo integrator ==
  in_1 : Inport
  Clock : Clock
      settings: Decimation=10
  Memory : Memory  Orientation=left  X0=init
  Memory1 : Memory
  Product : Product  SaturateOnIntegerOverflow=on  InputSameDT=on
  Sum : Sum  SaturateOnIntegerOverflow=on  InputSameDT=on
  Sum1 : Sum  Inputs=+-  SaturateOnIntegerOverflow=on  InputSameDT=on
  module : Fcn  Expr=rem(u[1],modu)
  out_1 : Outport  InitialOutput=0
  wires:
  module/1 -> Memory/1, out_1/1
  Sum/1 -> module/1
  Product/1 -> Sum/1
  Memory/1 -> Sum/2
  Sum1/1 -> Product/2
  in_1/1 -> Product/1
  Clock/1 -> Sum1/1, Memory1/1
  Memory1/1 -> Sum1/2

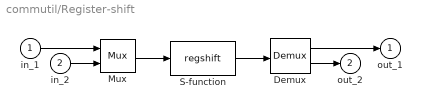
== system commutil/Register-shift ==
  in_1 : Inport
  in_2 : Inport  Port=2
  Demux : Demux  Outputs=[len_rg, 1]
  Mux : Mux  Inputs=2
  S-function : S-Function  FunctionName=regshift  Parameters=shft_out, thrhld
  out_1 : Outport  InitialOutput=0
  out_2 : Outport  Port=2  InitialOutput=0
  wires:
  in_2/1 -> Mux/2
  in_1/1 -> Mux/1
  Mux/1 -> S-function/1
  Demux/2 -> out_2/1
  Demux/1 -> out_1/1
  S-function/1 -> Demux/1

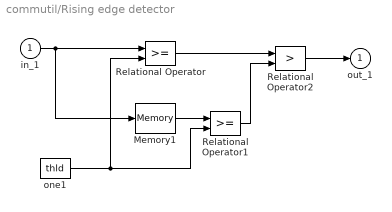
== system commutil/Rising edge detector ==
  in_1 : Inport
  Memory1 : Memory
  Relational Operator : RelationalOperator  InputSameDT=on
  Relational Operator1 : RelationalOperator  InputSameDT=on
  Relational Operator2 : RelationalOperator  Operator=>  InputSameDT=on
  one1 : Constant  Value=thld
  out_1 : Outport  InitialOutput=0
  wires:
  in_1/1 -> Memory1/1, Relational Operator/1
  Memory1/1 -> Relational Operator1/1
  one1/1 -> Relational Operator1/2, Relational Operator/2
  Relational Operator/1 -> Relational Operator2/1
  Relational Operator1/1 -> Relational Operator2/2
  Relational Operator2/1 -> out_1/1

== system commutil/Scheduled reset-int ==
  In1 : Inport
  Scheduled reset-int : S-Function  FunctionName=schdint  Parameters=td, ts, limit
  Out1 : Outport  InitialOutput=0
  wires:
  In1/1 -> Scheduled reset-int/1
  Scheduled reset-int/1 -> Out1/1

== system commutil/Scrambler ==
  In1 : Inport
  In2 : Inport  Port=2
  Demux : Demux  Outputs=[1 s]
  Mux : Mux  Inputs=2
  S-Function : S-Function  FunctionName=simscram  Parameters=M, poly, 0, ini_sta
  Out2 : Outport  InitialOutput=0
  Out3 : Outport  Port=2  InitialOutput=0
  wires:
  In1/1 -> Mux/1
  In2/1 -> Mux/2
  Mux/1 -> S-Function/1
  S-Function/1 -> Demux/1
  Demux/1 -> Out2/1
  Demux/2 -> Out3/1

== system commutil/Signal switch ==
  in_1 : Inport
  in_2 : Inport  Port=2
  Mux : Mux  Inputs=2
  S-function : S-Function  FunctionName=switchbx  Parameters=sw,df
  out_1 : Outport  InitialOutput=0
  wires:
  S-function/1 -> out_1/1
  Mux/1 -> S-function/1
  in_2/1 -> Mux/2
  in_1/1 -> Mux/1

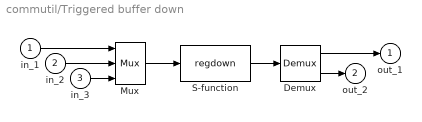
== system commutil/Triggered buffer down ==
  in_1 : Inport
  in_2 : Inport  Port=2
  in_3 : Inport  Port=3
  Demux : Demux  Outputs=[out_size 1]
  Mux : Mux  Inputs=[in_size 1 1]
  S-function : S-Function  FunctionName=regdown  Parameters=ini_idx, idx_inc, thrshld, cycl_flag
  out_1 : Outport  InitialOutput=0
  out_2 : Outport  Port=2  InitialOutput=0
  wires:
  S-function/1 -> Demux/1
  Mux/1 -> S-function/1
  in_1/1 -> Mux/1
  in_2/1 -> Mux/2
  in_3/1 -> Mux/3
  Demux/1 -> out_1/1
  Demux/2 -> out_2/1

== system commutil/Triggered signal switch ==
  in_1 : Inport
  in_2 : Inport  Port=2
  Mux : Mux  Inputs=2
  S-function : S-Function  FunctionName=stdmamux  Parameters=sw,ke,in,tt
  out_1 : Outport  InitialOutput=0
  wires:
  in_1/1 -> Mux/1
  in_2/1 -> Mux/2
  Mux/1 -> S-function/1
  S-function/1 -> out_1/1

== system commutil/Voltage-controlled oscillator ==
  in_1 : Inport
  Carrier frequency : Constant  Value=Fc
  Modulo integrator : commutil/Modulo integrator  modu=1  init=0
  Sensitivity : Gain  Gain=Kc  SaturateOnIntegerOverflow=on
  Sum : Sum  SaturateOnIntegerOverflow=on  InputSameDT=on
  sin : Fcn  Expr=Ac*sin(u[1]*pi2+Ph)
  out_1 : Outport  InitialOutput=0
  wires:
  Sum/1 -> Modulo integrator/1
  Modulo integrator/1 -> sin/1
  sin/1 -> out_1/1
  Carrier frequency/1 -> Sum/2
  Sensitivity/1 -> Sum/1
  in_1/1 -> Sensitivity/1

== system commutil/Counter/Accumulator ==
  " " : Inport
  Enable : EnablePort  StatesWhenEnabling=reset
  Trigger : TriggerPort
  Direct-Form II Transpose Filter : dsparch2/Direct-Form II Transpose Filter  num=1  den=[1 -1]  ic=0  frame=off  numCHANS=1
  "  " : Outport  OutputWhenDisabled=reset  InitialOutput=0
  wires:
  " "/1 -> Direct-Form II Transpose Filter/1
  Direct-Form II Transpose Filter/1 -> "  "/1

== system commutil/Data Mapper/Lookup ==
  In : Inport
  Enable : EnablePort
  Look-Up Table : Lookup  InputValues=IPValues  OutputValues=OPValues  SaturateOnIntegerOverflow=on
  Rounding Function : Rounding  Operator=round
  Saturation : Saturate  UpperLimit=SatValue  LowerLimit=0
  Out : Outport
  wires:
  Rounding Function/1 -> Look-Up Table/1
  Saturation/1 -> Rounding Function/1
  Look-Up Table/1 -> Out/1
  In/1 -> Saturation/1

== system commutil/Data Mapper/Straight ==
  In : Inport
  Enable : EnablePort
  Out : Outport
  wires:
  In/1 -> Out/1
